simulink model "Env_Unit"  (R2020b)
settings: configuration reference "gen_config" (kept outside this file)
undefined symbols (not defined in the file): Ts
libraries: simulink_extras x1
settings Model: DataDictionary=Hybrid_vehicle.sldd  SimulationMode=accelerator  Creator=Georg  LastModifiedBy=jy
settings ConfigSetRef: SourceName=gen_config

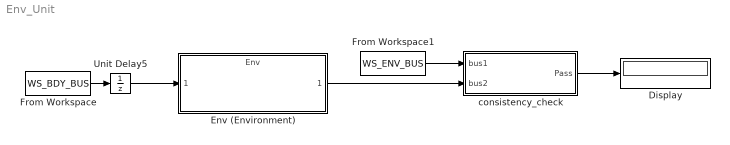
== system Env_Unit ==
  Display : Display
  Env (Environment) : ModelReference  ModelNameDialog=Env  SimulationMode=Normal  ModelReferenceVersion=2.20
  From Workspace : FromWorkspace  VariableName=WS_BDY_BUS  OutDataTypeStr=Bus: BDY_BUS  SampleTime=Ts  Interpolate=off  OutputAfterFinalValue=Holding final value
  From Workspace1 : FromWorkspace  VariableName=WS_ENV_BUS  OutDataTypeStr=Bus: ENV_BUS  SampleTime=Ts  Interpolate=off  OutputAfterFinalValue=Holding final value
  Unit Delay5 : UnitDelay  SampleTime=-1  HasFrameUpgradeWarning=on
  consistency_check : Subsystem
  wires:
  Env (Environment)/1 -> consistency_check/2(bus2)
  From Workspace/1 -> Unit Delay5/1
  Unit Delay5/1 -> Env (Environment)/1
  From Workspace1/1 -> consistency_check/1(bus1)
  consistency_check/1(Pass) -> Display/1

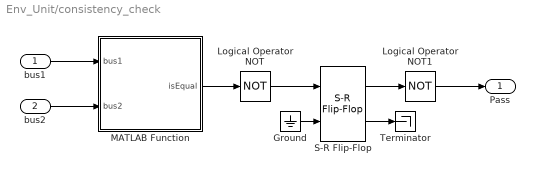
== system Env_Unit/consistency_check ==
  bus1 : Inport
  bus2 : Inport  Port=2
  Ground : Ground
  Logical Operator NOT : Logic  Operator=NOT  AllPortsSameDT=off  OutDataTypeStr=boolean
  Logical Operator NOT1 : Logic  Operator=NOT  AllPortsSameDT=off  OutDataTypeStr=boolean
  MATLAB Function : MATLAB Function  TreatAsAtomicUnit=on
  S-R Flip-Flop : simulink_extras/Flip Flops/S-R Flip-Flop  initial_condition=0
  Terminator : Terminator
  Pass : Outport  VectorParamsAs1DForOutWhenUnconnected=off
  wires:
  bus1/1 -> MATLAB Function/1(bus1)
  bus2/1 -> MATLAB Function/2(bus2)
  MATLAB Function/1(isEqual) -> Logical Operator NOT/1
  Logical Operator NOT/1 -> S-R Flip-Flop/1
  Ground/1 -> S-R Flip-Flop/2
  S-R Flip-Flop/2 -> Terminator/1
  S-R Flip-Flop/1 -> Logical Operator NOT1/1
  Logical Operator NOT1/1 -> Pass/1

== matlab function Env_Unit/consistency_check/MATLAB Function ==
  data: bus1 input; isEqual output; bus2 input
function isEqual = fcn(bus1, bus2)
isEqual = isequal(bus1, bus2);
